simulink model "HevMmPowertrainController"  (R2024a)
settings: configuration reference "VehicleFixed10ms" (kept outside this file)
undefined symbols (not defined in the file): CtrlBcuTrlrBrkGain, CtrlVcuHevMmBattChrgPwrMax, CtrlVcuHevMmBattDischrgPwrMax, CtrlVcuHevMmChrgLmtBpt, CtrlVcuHevMmCSChrgFctr, CtrlVcuHevMmDischrgLmtBpt, CtrlVcuHevMmEngPwr, CtrlVcuHevMmEngSpd, CtrlVcuHevMmEngTrq, CtrlVcuHevMmN_idle, CtrlVcuHevMmRegenBrkCutOff, CtrlVcuHevMmRegenBrkSpdBpt, CtrlVcuHevMmSocBpt, CtrlVcuHevMmSOCChrgFctr, CtrlVcuHevMmSOCmax, CtrlVcuHevMmSOCmin, CtrlVcuHevMmSOCtarget, DiscIntNeverNeededParam, PlntBattChrgMax, PlntBrkActrBoreFrnt, PlntBrkFrntBias, PlntBrkKinFricCffFrnt, PlntBrkNumPadsFrnt, PlntBrkPadMeanRadiusFrnt, PlntBrkPrsFctr, PlntBrkRearBias, PlntDiffrntlRatio, PlntEM1EffTbl, PlntEM1Spd, PlntEM1SpdEff, PlntEM1Trq, PlntEM1TrqEff, PlntEM2EffTbl, PlntEM2Spd, PlntEM2SpdEff, PlntEM2Trq, PlntEM2TrqEff, PlntHevMmGenGearRatio, PlntHevMmMotGearRatio, PlntVehMass, PlntWhlLdRadius
libraries: simulink x15, autolibutils x1
(part 1 of 2)
settings Model: DataDictionary=VirtualVehicleTemplate.sldd  ModifiedByFormat=The MathWorks, Inc.  Creator=The MathWorks, Inc.  LastModifiedBy=The MathWorks, Inc.
settings ConfigSetRef: SourceName=VehicleFixed10ms

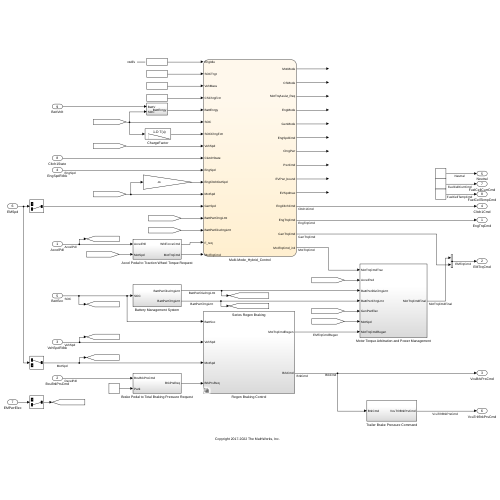
[thumbnail: Simulink's stored preview of the top-level diagram]
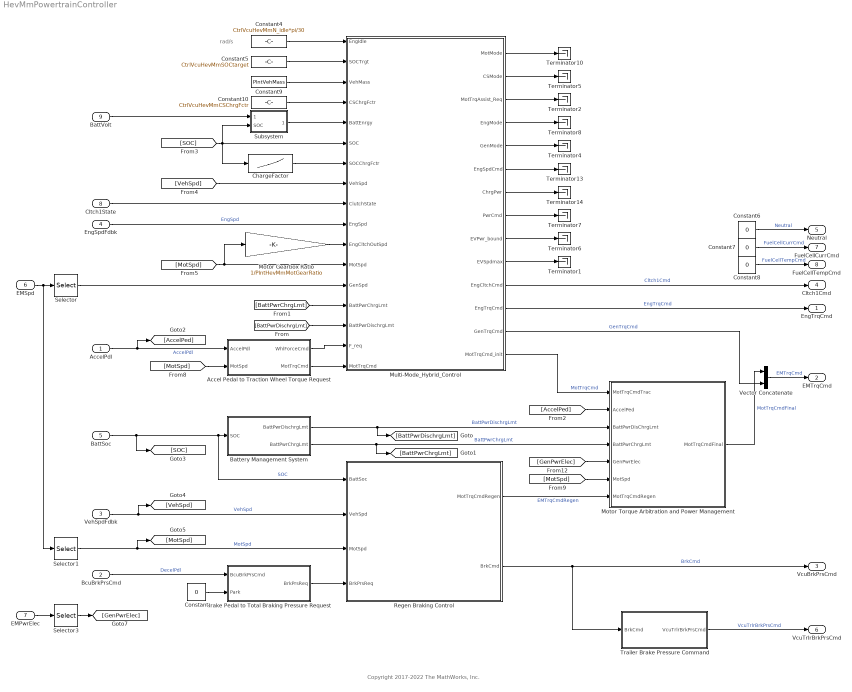
== system HevMmPowertrainController ==
  note: rad/s
  note: Copyright 2017-2022 The MathWorks, Inc.
  AccelPdl : Inport  OutDataTypeStr=double  PortDimensions=1
  BcuBrkPrsCmd : Inport  Port=2  OutDataTypeStr=double  PortDimensions=4
  VehSpdFdbk : Inport  Port=3  OutDataTypeStr=double  PortDimensions=1
  EngSpdFdbk : Inport  Port=4  OutDataTypeStr=double  PortDimensions=1
  BattSoc : Inport  Port=5  OutDataTypeStr=double  PortDimensions=1
  EMSpd : Inport  Port=6  OutDataTypeStr=double  PortDimensions=2
  EMPwrElec : Inport  Port=7  OutDataTypeStr=double  PortDimensions=2
  Cltch1State : Inport  Port=8  OutDataTypeStr=boolean  PortDimensions=1
  BattVolt : Inport  Port=9  OutDataTypeStr=double  PortDimensions=1
  Accel Pedal to Traction Wheel Torque Request : Subsystem  InitFcn=[~]=autosharedicon('autolibinternalvvblock',gcb,0);
  Battery Management System : Subsystem
  Brake Pedal to Total Braking Pressure Request : Subsystem
  ChargeFactor : Lookup_n-D  NumberOfTableDimensions=1  BreakpointsForDimension1=[CtrlVcuHevMmSOCmin CtrlVcuHevMmSOCtarget CtrlVcuHevMmSOCmax]  Table=CtrlVcuHevMmSOCChrgFctr  ExtrapMethod=Clip  UseLastTableValue=on  InternalRulePriority=Speed  RndMeth=Simplest
  Constant{,6..8} (4 alike) : Constant  Value=0  SampleTime=-1
  Constant10 : Constant  Value=CtrlVcuHevMmCSChrgFctr  SampleTime=-1
  Constant4 : Constant  Value=CtrlVcuHevMmN_idle*pi/30  SampleTime=-1
  Constant5 : Constant  Value=CtrlVcuHevMmSOCtarget  SampleTime=-1
  Constant9 : Constant  Value=PlntVehMass  SampleTime=-1
  Motor Gearbox Ratio : Gain  Gain=1/PlntHevMmMotGearRatio
  Motor Torque Arbitration and Power Management : Subsystem
  Multi-Mode_Hybrid_Control : Stateflow chart  TreatAsAtomicUnit=on
  Regen Braking Control : Subsystem  Variant=on  VariantControlMode=label  VariantControl=(default)  LabelModeActiveChoice=Variant
  Selector : Selector  InputPortWidth=2  IndexOptions=Index vector (dialog)  Indices=[2]  OutputSizes=1
  Selector1 : Selector  InputPortWidth=2  IndexOptions=Index vector (dialog)  Indices=[1]  OutputSizes=1
  Selector3 : Selector  InputPortWidth=2  IndexOptions=Index vector (dialog)  Indices=[2]  OutputSizes=1
  Subsystem : Subsystem
  Terminator{1..2,4..8,10,13..14} (10 alike) : Terminator
  Trailer Brake Pressure Command : Subsystem
  Vector Concatenate : Concatenate
  EngTrqCmd : Outport  OutDataTypeStr=double  PortDimensions=1  VectorParamsAs1DForOutWhenUnconnected=off
  EMTrqCmd : Outport  Port=2  OutDataTypeStr=double  PortDimensions=2  VectorParamsAs1DForOutWhenUnconnected=off
  VcuBrkPrsCmd : Outport  Port=3  OutDataTypeStr=double  PortDimensions=4  VectorParamsAs1DForOutWhenUnconnected=off
  Cltch1Cmd : Outport  Port=4  OutDataTypeStr=double  PortDimensions=1  VectorParamsAs1DForOutWhenUnconnected=off
  Neutral : Outport  Port=5  OutDataTypeStr=double  PortDimensions=1  VectorParamsAs1DForOutWhenUnconnected=off
  VcuTrlrBrkPrsCmd : Outport  Port=6  PortDimensions=6  VectorParamsAs1DForOutWhenUnconnected=off
  FuelCellCurrCmd : Outport  Port=7  OutDataTypeStr=double  PortDimensions=1
  FuelCellTempCmd : Outport  Port=8  OutDataTypeStr=double  PortDimensions=1
  wires:
  AccelPdl/1 -> Accel Pedal to Traction Wheel Torque Request/1(AccelPdl), [AccelPed]  "AccelPdl"
  BcuBrkPrsCmd/1 -> Brake Pedal to Total Braking Pressure Request/1(BcuBrkPrsCmd)  "DecelPdl"
  VehSpdFdbk/1 -> [VehSpd], Regen Braking Control/2("VehSpd ")  "VehSpd"
  EngSpdFdbk/1 -> Multi-Mode_Hybrid_Control/10(EngSpd)  "EngSpd"
  BattSoc/1 -> [SOC], Regen Braking Control/1("BattSoc "), Battery Management System/1(SOC)  "SOC"
  Selector1/1 -> [MotSpd], Regen Braking Control/3("MotSpd ")  "MotSpd"
  Battery Management System/2(BattPwrChrgLmt) -> [BattPwrChrgLmt], Motor Torque Arbitration and Power Management/4("BattPwrChrgLmt ")  "BattPwrChrgLmt"
  Battery Management System/1(BattPwrDischrgLmt) -> Motor Torque Arbitration and Power Management/3(BattPwrDisChrgLmt), [BattPwrDischrgLmt]  "BattPwrDischrgLmt"
  [SOC] -> ChargeFactor/1, Subsystem/2(SOC), Multi-Mode_Hybrid_Control/6(SOC)
  [VehSpd] -> Multi-Mode_Hybrid_Control/8(VehSpd)
  Constant4/1 -> Multi-Mode_Hybrid_Control/1(EngIdle)
  Multi-Mode_Hybrid_Control/14(MotTrqCmd_init) -> Motor Torque Arbitration and Power Management/1(MotTrqCmdTrac)  "MotTrqCmd"
  Brake Pedal to Total Braking Pressure Request/1(BrkPrsReq) -> Regen Braking Control/4("BrkPrsReq ")
  Regen Braking Control/1(" MotTrqCmdRegen") -> Motor Torque Arbitration and Power Management/7(MotTrqCmdRegen)  "EMTrqCmdRegen"
  Constant5/1 -> Multi-Mode_Hybrid_Control/2(SOCTrgt)
  ChargeFactor/1 -> Multi-Mode_Hybrid_Control/7(SOCChrgFctr)
  [MotSpd] -> Accel Pedal to Traction Wheel Torque Request/2(MotSpd)
  [AccelPed] -> Motor Torque Arbitration and Power Management/2(AccelPed)
  Selector/1 -> Multi-Mode_Hybrid_Control/13(GenSpd)
  Selector3/1 -> [GenPwrElec]
  EMPwrElec/1 -> Selector3/1
  Motor Torque Arbitration and Power Management/1(MotTrqCmdFinal) -> Vector Concatenate/1  "MotTrqCmdFinal"
  Multi-Mode_Hybrid_Control/13(GenTrqCmd) -> Vector Concatenate/2  "GenTrqCmd"
  Multi-Mode_Hybrid_Control/12(EngTrqCmd) -> EngTrqCmd/1  "EngTrqCmd"
  Constant/1 -> Brake Pedal to Total Braking Pressure Request/2(Park)
  [MotSpd] -> Motor Torque Arbitration and Power Management/6(MotSpd)
  [GenPwrElec] -> Motor Torque Arbitration and Power Management/5(GenPwrElec)
  Vector Concatenate/1 -> EMTrqCmd/1  "EMTrqCmd"
  EMSpd/1 -> Selector1/1, Selector/1
  Constant6/1 -> Neutral/1  "Neutral"
  Multi-Mode_Hybrid_Control/11(EngCltchCmd) -> Cltch1Cmd/1  "Cltch1Cmd"
  Constant7/1 -> FuelCellCurrCmd/1  "FuelCellCurrCmd"
  Constant8/1 -> FuelCellTempCmd/1  "FuelCellTempCmd"
  Multi-Mode_Hybrid_Control/7(ChrgPwr) -> Terminator14/1
  Multi-Mode_Hybrid_Control/8(PwrCmd) -> Terminator7/1
  Multi-Mode_Hybrid_Control/9(EVPwr_bound) -> Terminator6/1
  Multi-Mode_Hybrid_Control/10(EVSpdmax) -> Terminator1/1
  Multi-Mode_Hybrid_Control/6(EngSpdCmd) -> Terminator13/1
  Multi-Mode_Hybrid_Control/5(GenMode) -> Terminator4/1
  Multi-Mode_Hybrid_Control/4(EngMode) -> Terminator8/1
  Multi-Mode_Hybrid_Control/3(MotTrqAssist_Req) -> Terminator2/1
  Multi-Mode_Hybrid_Control/2(CSMode) -> Terminator5/1
  Multi-Mode_Hybrid_Control/1(MotMode) -> Terminator10/1
  [BattPwrChrgLmt] -> Multi-Mode_Hybrid_Control/14(BattPwrChrgLmt)
  [BattPwrDischrgLmt] -> Multi-Mode_Hybrid_Control/15(BattPwrDischrgLmt)
  [MotSpd] -> Motor Gearbox Ratio/1, Multi-Mode_Hybrid_Control/12(MotSpd)
  Cltch1State/1 -> Multi-Mode_Hybrid_Control/9(ClutchState)
  Motor Gearbox Ratio/1 -> Multi-Mode_Hybrid_Control/11(EngCltchOutSpd)
  Constant9/1 -> Multi-Mode_Hybrid_Control/3(VehMass)
  Constant10/1 -> Multi-Mode_Hybrid_Control/4(CSChrgFctr)
  Subsystem/1(BattEnrgy) -> Multi-Mode_Hybrid_Control/5(BattEnrgy)
  BattVolt/1 -> Subsystem/1(BattV)
  Accel Pedal to Traction Wheel Torque Request/2(MotTrqCmd) -> Multi-Mode_Hybrid_Control/17(MotTrqCmd)
  Accel Pedal to Traction Wheel Torque Request/1(WhlForceCmd) -> Multi-Mode_Hybrid_Control/16(F_req)
  Regen Braking Control/2(" BrkCmd") -> Trailer Brake Pressure Command/1(BrkCmd), VcuBrkPrsCmd/1  "BrkCmd"
  Trailer Brake Pressure Command/1(VcuTrlrBrkPrsCmd) -> VcuTrlrBrkPrsCmd/1  "VcuTrlrBrkPrsCmd"

== system HevMmPowertrainController/Accel Pedal to Traction Wheel Torque Request ==
  AccelPdl : Inport
  MotSpd : Inport  Port=2
  MaxMotTrqVsSpd : Lookup_n-D  NumberOfTableDimensions=1  BreakpointsForDimension1=PlntEM1Spd*30/pi  Table=PlntEM1Trq  ExtrapMethod=Clip  UseLastTableValue=on  InternalRulePriority=Speed  OutDataTypeStr=Inherit: Inherit from 'Table data'  RndMeth=Simplest
  MotTrq_to_WhlForce : Gain  Gain=(PlntDiffrntlRatio*PlntHevMmMotGearRatio)/PlntWhlLdRadius
  Product1 : Product
  rads_to_rpm : Gain  Gain=30/pi
  WhlForceCmd : Outport  VectorParamsAs1DForOutWhenUnconnected=off
  MotTrqCmd : Outport  Port=2  VectorParamsAs1DForOutWhenUnconnected=off
  wires:
  Product1/1 -> MotTrqCmd/1, MotTrq_to_WhlForce/1
  MaxMotTrqVsSpd/1 -> Product1/2
  AccelPdl/1 -> Product1/1
  rads_to_rpm/1 -> MaxMotTrqVsSpd/1
  MotSpd/1 -> rads_to_rpm/1
  MotTrq_to_WhlForce/1 -> WhlForceCmd/1

== system HevMmPowertrainController/Battery Management System ==
  note: Limit battery charge / discharge power based on SOC
  SOC : Inport
  ChrgLmt : Lookup_n-D  NumberOfTableDimensions=1  BreakpointsForDimension1=CtrlVcuHevMmSocBpt  Table=CtrlVcuHevMmChrgLmtBpt  ExtrapMethod=Clip  UseLastTableValue=on  InternalRulePriority=Speed  RndMeth=Simplest
  DischrgLmt : Lookup_n-D  NumberOfTableDimensions=1  BreakpointsForDimension1=CtrlVcuHevMmSocBpt  Table=CtrlVcuHevMmDischrgLmtBpt  ExtrapMethod=Clip  UseLastTableValue=on  InternalRulePriority=Speed  RndMeth=Simplest
  MaxChrg : Constant  Value=CtrlVcuHevMmBattChrgPwrMax  SampleTime=-1
  MaxDischrg : Constant  Value=CtrlVcuHevMmBattDischrgPwrMax  SampleTime=-1
  Product : Product
  Product1 : Product
  BattPwrDischrgLmt : Outport  VectorParamsAs1DForOutWhenUnconnected=off
  BattPwrChrgLmt : Outport  Port=2  VectorParamsAs1DForOutWhenUnconnected=off
  wires:
  SOC/1 -> DischrgLmt/1, ChrgLmt/1
  MaxChrg/1 -> Product1/2
  MaxDischrg/1 -> Product/2
  Product/1 -> BattPwrDischrgLmt/1
  Product1/1 -> BattPwrChrgLmt/1
  ChrgLmt/1 -> Product1/1
  DischrgLmt/1 -> Product/1

== system HevMmPowertrainController/Brake Pedal to Total Braking Pressure Request ==
  BcuBrkPrsCmd : Inport
  Park : Inport  Port=2
  Front Bias : Constant  Value=PlntBrkFrntBias  SampleTime=-1
  Gain4 : Gain  Gain=PlntBrkPrsFctr
  Mux : Mux
  Product : Product
  Rear Bias : Constant  Value=PlntBrkRearBias  SampleTime=-1
  Terminator : Terminator
  BrkPrsReq : Outport  VectorParamsAs1DForOutWhenUnconnected=off
  wires:
  BcuBrkPrsCmd/1 -> Product/2
  Mux/1 -> Product/1
  Rear Bias/1 -> Mux/4, Mux/3
  Front Bias/1 -> Mux/1, Mux/2
  Gain4/1 -> BrkPrsReq/1
  Product/1 -> Gain4/1
  Park/1 -> Terminator/1

== system HevMmPowertrainController/Motor Torque Arbitration and Power Management ==
  MotTrqCmdTrac : Inport
  AccelPed : Inport  Port=2
  BattPwrDisChrgLmt : Inport  Port=3
  "BattPwrChrgLmt " : Inport  Port=4
  GenPwrElec : Inport  Port=5
  MotSpd : Inport  Port=6
  MotTrqCmdRegen : Inport  Port=7
  Accel Decel Switch : Switch  Criteria=u2 > Threshold  SaturateOnIntegerOverflow=off  InputSameDT=off
  Compare To Constant : simulink/Logic and Bit Operations/Compare To Constant  relop=>  const=0  OutDataTypeStr=boolean
  Power Management : Subsystem
  MotTrqCmdFinal : Outport  VectorParamsAs1DForOutWhenUnconnected=off
  wires:
  AccelPed/1 -> Compare To Constant/1
  MotTrqCmdRegen/1 -> Accel Decel Switch/3
  Compare To Constant/1 -> Accel Decel Switch/2
  MotTrqCmdTrac/1 -> Accel Decel Switch/1
  Power Management/1(MotTrqLim) -> MotTrqCmdFinal/1
  Accel Decel Switch/1 -> Power Management/5(MotTrqCmd)
  BattPwrDisChrgLmt/1 -> Power Management/1(BattPwrDischrgLmt)
  GenPwrElec/1 -> Power Management/2(GenPwrElec)
  "BattPwrChrgLmt "/1 -> Power Management/3(BattPwrChrgLmt)
  MotSpd/1 -> Power Management/4(MotSpd)

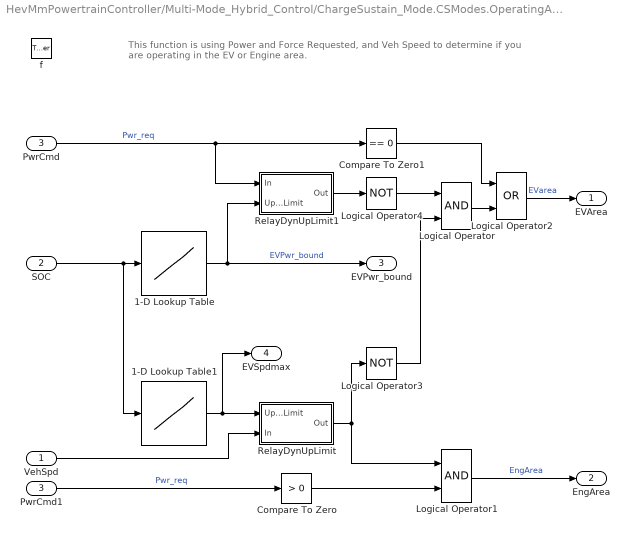
== system HevMmPowertrainController/Multi-Mode_Hybrid_Control/ChargeSustain_Mode.CSModes.OperatingAreaCalc ==
  note: This function is using Power and Force Requested, and Veh Speed to determine
      | if you are operating in the EV or Engine area.
  VehSpd : Inport  PortDimensions=1
  SOC : Inport  Port=2  PortDimensions=1
  PwrCmd : Inport  Port=3
  f : TriggerPort  TriggerType=function-call  VariantControl=Variant  StatesWhenEnabling=reset
      settings: CopyFcn=Stateflow.SLINSF.SimulinkMan.removeBlockPreDeleteFcn  PreDeleteFcn=Stateflow.SLINSF.SimulinkMan.unsafePredeleteFcn
  1-D Lookup Table : Lookup_n-D  NumberOfTableDimensions=1  BreakpointsForDimension1=[CtrlVcuHevMmSOCmin CtrlVcuHevMmSOCtarget CtrlVcuHevMmSOCmax]  Table=[0 CtrlVcuHevMmEngPwr(4) CtrlVcuHevMmBattDischrgPwrMax]  ExtrapMethod=Clip  UseLastTableValue=on  InternalRulePriority=Speed  RndMeth=Simplest
  1-D Lookup Table1 : Lookup_n-D  NumberOfTableDimensions=1  BreakpointsForDimension1=[CtrlVcuHevMmSOCtarget CtrlVcuHevMmSOCmax]  Table=[24.6 33.5]  ExtrapMethod=Clip  UseLastTableValue=on  InternalRulePriority=Speed  RndMeth=Simplest
  Compare To Zero : simulink/Logic and Bit Operations/Compare To Zero  relop=>  OutDataTypeStr=boolean
  Compare To Zero1 : simulink/Logic and Bit Operations/Compare To Zero  relop===  OutDataTypeStr=boolean
  Logical Operator : Logic  AllPortsSameDT=off  OutDataTypeStr=boolean
  Logical Operator1 : Logic  AllPortsSameDT=off  OutDataTypeStr=boolean
  Logical Operator2 : Logic  Operator=OR  AllPortsSameDT=off  OutDataTypeStr=boolean
  Logical Operator3 : Logic  Operator=NOT  AllPortsSameDT=off  OutDataTypeStr=boolean
  Logical Operator4 : Logic  Operator=NOT  AllPortsSameDT=off  OutDataTypeStr=boolean
  PwrCmd1 : InportShadow  Port=3
  RelayDynUpLimit : Subsystem
  RelayDynUpLimit1 : Subsystem
  EVArea : Outport  VectorParamsAs1DForOutWhenUnconnected=off
  EngArea : Outport  Port=2  VectorParamsAs1DForOutWhenUnconnected=off
  EVPwr_bound : Outport  Port=3  VectorParamsAs1DForOutWhenUnconnected=off
  EVSpdmax : Outport  Port=4  VectorParamsAs1DForOutWhenUnconnected=off
  wires:
  Logical Operator1/1 -> EngArea/1  "EngArea"
  Logical Operator/1 -> Logical Operator2/2
  Logical Operator3/1 -> Logical Operator/2
  VehSpd/1 -> RelayDynUpLimit/2(In)
  1-D Lookup Table1/1 -> EVSpdmax/1, RelayDynUpLimit/1(Upper Limit)
  PwrCmd/1 -> RelayDynUpLimit1/1(In), Compare To Zero1/1  "Pwr_req"
  Compare To Zero1/1 -> Logical Operator2/1
  Logical Operator2/1 -> EVArea/1  "EVarea"
  1-D Lookup Table/1 -> RelayDynUpLimit1/2(Upper Limit), EVPwr_bound/1  "EVPwr_bound"
  SOC/1 -> 1-D Lookup Table/1, 1-D Lookup Table1/1
  Compare To Zero/1 -> Logical Operator1/2
  PwrCmd1/1 -> Compare To Zero/1  "Pwr_req"
  RelayDynUpLimit/1(Out) -> Logical Operator1/1, Logical Operator3/1
  RelayDynUpLimit1/1(Out) -> Logical Operator4/1
  Logical Operator4/1 -> Logical Operator/1

== system HevMmPowertrainController/Multi-Mode_Hybrid_Control/ChargeSustain_Mode.Engine_Control.Eng.Clutch_Close.ClutchControl ==
  note: When error is <=5 rads/s
      | clutch commanded closed
  EngCltchOutSpd : Inport
  EngSpd : Inport  Port=2
  f : TriggerPort  TriggerType=function-call  VariantControl=Variant  StatesWhenEnabling=reset  SampleTime=-1
      settings: CopyFcn=Stateflow.SLINSF.SimulinkMan.removeBlockPreDeleteFcn  PreDeleteFcn=Stateflow.SLINSF.SimulinkMan.unsafePredeleteFcn
  Abs1 : Abs  SaturateOnIntegerOverflow=off
  Compare To Constant1 : simulink/Logic and Bit Operations/Compare To Constant  relop=<=  const=5  OutDataTypeStr=boolean
  Subtract2 : Sum  Inputs=+-
  EngCltchCmd : Outport  VectorParamsAs1DForOutWhenUnconnected=off
  wires:
  EngCltchOutSpd/1 -> Subtract2/1
  Abs1/1 -> Compare To Constant1/1
  EngSpd/1 -> Subtract2/2
  Subtract2/1 -> Abs1/1
  Compare To Constant1/1 -> EngCltchCmd/1

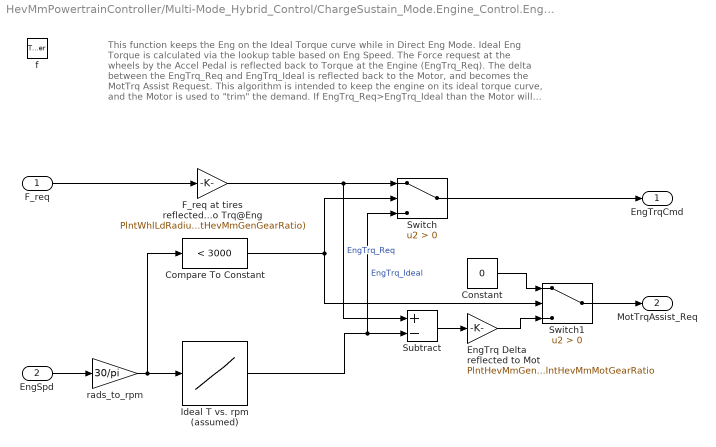
== system HevMmPowertrainController/Multi-Mode_Hybrid_Control/ChargeSustain_Mode.Engine_Control.Eng.Direct_Engine_Drive.EngTrqControl ==
  note: This function keeps the Eng on the Ideal Torque curve while in Direct Eng Mode.
      | Ideal Eng Torque is calculated via the lookup table based on Eng Speed.
      | The Force request at the wheels by the Accel Pedal is reflected back to Torque at
      | the Engine (EngTrq_Req).  The delta between the EngTrq_Req and EngTrq_Ideal
      | is reflected back to the Motor, and becomes the MotTrq Assist Request.  This algorithm
      | is intended to keep the engine on its ideal torque curve, and the Motor is used to "trim"
      | the demand.  If EngTrq_Req>EngTrq_Ideal than the Motor will provide assistance in
      | traction.  If EngTrq_Req<EngTrq_Ideal, the Motor will provide assistance through regen.
  F_req : Inport
  EngSpd : Inport  Port=2
  f : TriggerPort  TriggerType=function-call  VariantControl=Variant  StatesWhenEnabling=reset  SampleTime=-1
      settings: CopyFcn=Stateflow.SLINSF.SimulinkMan.removeBlockPreDeleteFcn  PreDeleteFcn=Stateflow.SLINSF.SimulinkMan.unsafePredeleteFcn
  Compare To Constant : simulink/Logic and Bit Operations/Compare To Constant  relop=<  const=3000  OutDataTypeStr=boolean
  Constant : Constant  Value=0  SampleTime=-1
  EngTrq Delta reflected to Mot : Gain  Gain=PlntHevMmGenGearRatio/PlntHevMmMotGearRatio
  F_req at tires reflected back to Trq@Eng : Gain  Gain=PlntWhlLdRadius/(PlntDiffrntlRatio*PlntHevMmGenGearRatio)
  Ideal T vs. rpm (assumed) : Lookup_n-D  NumberOfTableDimensions=1  BreakpointsForDimension1=CtrlVcuHevMmEngSpd  BreakpointsForDimension1DataTypeStr=Inherit: Inherit from 'Breakpoint data'  Table=CtrlVcuHevMmEngTrq  TableDataTypeStr=Inherit: Inherit from 'Table data'  ExtrapMethod=Clip  UseLastTableValue=on  InternalRulePriority=Speed  OutDataTypeStr=single  RndMeth=Simplest
  Subtract : Sum  Inputs=+-
  Switch : Switch  Criteria=u2 > Threshold  SaturateOnIntegerOverflow=off  InputSameDT=off
  Switch1 : Switch  Criteria=u2 > Threshold  SaturateOnIntegerOverflow=off  InputSameDT=off
  rads_to_rpm : Gain  Gain=30/pi
  EngTrqCmd : Outport  VectorParamsAs1DForOutWhenUnconnected=off
  MotTrqAssist_Req : Outport  Port=2  VectorParamsAs1DForOutWhenUnconnected=off
  wires:
  F_req/1 -> F_req at tires reflected back to Trq@Eng/1
  F_req at tires reflected back to Trq@Eng/1 -> Switch/1, Subtract/1  "EngTrq_Req"
  Subtract/1 -> EngTrq Delta reflected to Mot/1
  Ideal T vs. rpm (assumed)/1 -> Subtract/2, Switch/3  "EngTrq_Ideal"
  rads_to_rpm/1 -> Compare To Constant/1, Ideal T vs. rpm (assumed)/1
  EngSpd/1 -> rads_to_rpm/1
  Compare To Constant/1 -> Switch1/2, Switch/2
  EngTrq Delta reflected to Mot/1 -> Switch1/3
  Constant/1 -> Switch1/1
  Switch/1 -> EngTrqCmd/1
  Switch1/1 -> MotTrqAssist_Req/1

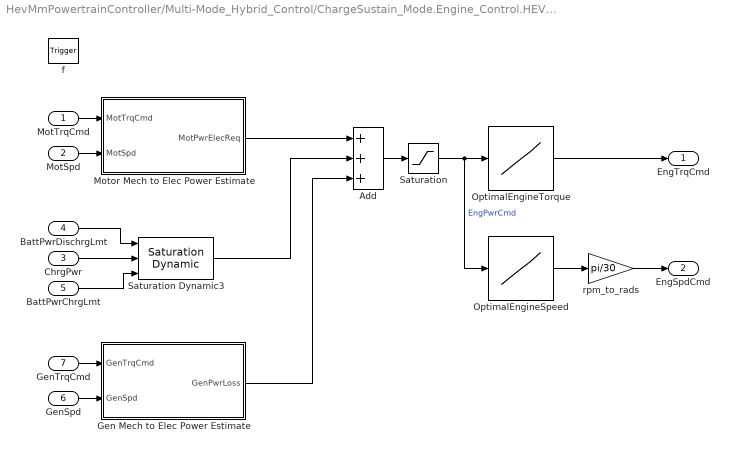
== system HevMmPowertrainController/Multi-Mode_Hybrid_Control/ChargeSustain_Mode.Engine_Control.HEV.TrqCalc ==
  MotTrqCmd : Inport
  MotSpd : Inport  Port=2
  ChrgPwr : Inport  Port=3
  BattPwrDischrgLmt : Inport  Port=4
  BattPwrChrgLmt : Inport  Port=5
  GenSpd : Inport  Port=6
  GenTrqCmd : Inport  Port=7
  f : TriggerPort  TriggerType=function-call  VariantControl=Variant  StatesWhenEnabling=reset
      settings: CopyFcn=Stateflow.SLINSF.SimulinkMan.removeBlockPreDeleteFcn  PreDeleteFcn=Stateflow.SLINSF.SimulinkMan.unsafePredeleteFcn
  Add : Sum  Inputs=+++
  Gen Mech to Elec Power Estimate : Subsystem
  Motor Mech to Elec Power Estimate : Subsystem
  OptimalEngineSpeed : Lookup_n-D  NumberOfTableDimensions=1  BreakpointsForDimension1=CtrlVcuHevMmEngPwr  Table=CtrlVcuHevMmEngSpd  ExtrapMethod=Clip  UseLastTableValue=on  InternalRulePriority=Speed  RndMeth=Simplest
  OptimalEngineTorque : Lookup_n-D  NumberOfTableDimensions=1  BreakpointsForDimension1=CtrlVcuHevMmEngPwr  Table=CtrlVcuHevMmEngTrq  ExtrapMethod=Clip  UseLastTableValue=on  InternalRulePriority=Speed  RndMeth=Simplest
  Saturation : Saturate  UpperLimit=inf  LowerLimit=0
  Saturation Dynamic3 : simulink/Discontinuities/Saturation Dynamic  OutMin=[]  OutMax=[]  OutDataTypeStr=Inherit: Same as second input  OutDataType=fixdt(1, 16)  OutScaling=2^-10  DoSatur=off
  rpm_to_rads : Gain  Gain=pi/30
  EngTrqCmd : Outport  VectorParamsAs1DForOutWhenUnconnected=off
  EngSpdCmd : Outport  Port=2  VectorParamsAs1DForOutWhenUnconnected=off
  wires:
  rpm_to_rads/1 -> EngSpdCmd/1
  OptimalEngineSpeed/1 -> rpm_to_rads/1
  Saturation/1 -> OptimalEngineTorque/1, OptimalEngineSpeed/1  "EngPwrCmd"
  MotTrqCmd/1 -> Motor Mech to Elec Power Estimate/1(MotTrqCmd)
  MotSpd/1 -> Motor Mech to Elec Power Estimate/2(MotSpd)
  Motor Mech to Elec Power Estimate/1(MotPwrElecReq) -> Add/1
  Add/1 -> Saturation/1
  ChrgPwr/1 -> Saturation Dynamic3/2
  BattPwrChrgLmt/1 -> Saturation Dynamic3/3
  Saturation Dynamic3/1 -> Add/2
  BattPwrDischrgLmt/1 -> Saturation Dynamic3/1
  OptimalEngineTorque/1 -> EngTrqCmd/1
  GenSpd/1 -> Gen Mech to Elec Power Estimate/2(GenSpd)
  GenTrqCmd/1 -> Gen Mech to Elec Power Estimate/1(GenTrqCmd)
  Gen Mech to Elec Power Estimate/1(GenPwrLoss) -> Add/3

== system HevMmPowertrainController/Multi-Mode_Hybrid_Control/ChargeSustain_Mode.Generator_Control.On.GenControl ==
  EngSpd : Inport
  EngSpdCmd : Inport  Port=2
  f : TriggerPort  TriggerType=function-call  VariantControl=Variant  StatesWhenEnabling=reset  SampleTime=-1
      settings: CopyFcn=Stateflow.SLINSF.SimulinkMan.removeBlockPreDeleteFcn  PreDeleteFcn=Stateflow.SLINSF.SimulinkMan.unsafePredeleteFcn
  State-Feedback Controller : Subsystem
  Torque Limit : Subsystem
  GenTrqCmd : Outport  VectorParamsAs1DForOutWhenUnconnected=off
  wires:
  EngSpd/1 -> State-Feedback Controller/2(y), Torque Limit/2(GenSpd)
  EngSpdCmd/1 -> State-Feedback Controller/1(r)
  Torque Limit/1(GenTrqCmd) -> GenTrqCmd/1
  State-Feedback Controller/1(Out1) -> Torque Limit/1(GenTrq)

== system HevMmPowertrainController/Regen Braking Control ==
  "BattSoc " : Inport
  "VehSpd " : Inport  Port=2
  "MotSpd " : Inport  Port=3
  "BrkPrsReq " : Inport  Port=4
  Parallel Regen Braking : Subsystem  InitFcn=[~]=autosharedicon('autolibinternalvvblock',gcb,0);  VariantControl=(default)
  Series Regen Braking : Subsystem  InitFcn=[~]=autosharedicon('autolibinternalvvblock',gcb,0);  VariantControl=Variant
  " MotTrqCmdRegen" : Outport  VectorParamsAs1DForOutWhenUnconnected=off
  " BrkCmd" : Outport  Port=2  VectorParamsAs1DForOutWhenUnconnected=off

== system HevMmPowertrainController/Subsystem ==
  BattV : Inport
  SOC : Inport  Port=2
  BattCap_As : Constant  Value=PlntBattChrgMax*3600  SampleTime=-1
  Gain1 : Gain  Gain=1/100
  Product : Product  Inputs=3
  BattEnrgy : Outport  VectorParamsAs1DForOutWhenUnconnected=off
  wires:
  SOC/1 -> Gain1/1
  BattCap_As/1 -> Product/1
  Product/1 -> BattEnrgy/1
  BattV/1 -> Product/2
  Gain1/1 -> Product/3

== system HevMmPowertrainController/Trailer Brake Pressure Command ==
  BrkCmd : Inport
  Gain1 : Gain  Gain=CtrlBcuTrlrBrkGain
  Probe : Probe  ProbeSampleTime=off  ProbeComplexSignal=off
  Product : Product  Inputs=*/
  Selector2 : Selector  InputPortWidth=1  IndexOptions=Index vector (dialog)  Indices=[1 1 1 1 1 1]  OutputSizes=1
  Sum : Sum  Inputs=+
  VcuTrlrBrkPrsCmd : Outport
  wires:
  Gain1/1 -> Selector2/1
  Product/1 -> Gain1/1
  Probe/1 -> Product/2
  BrkCmd/1 -> Probe/1, Sum/1
  Sum/1 -> Product/1
  Selector2/1 -> VcuTrlrBrkPrsCmd/1

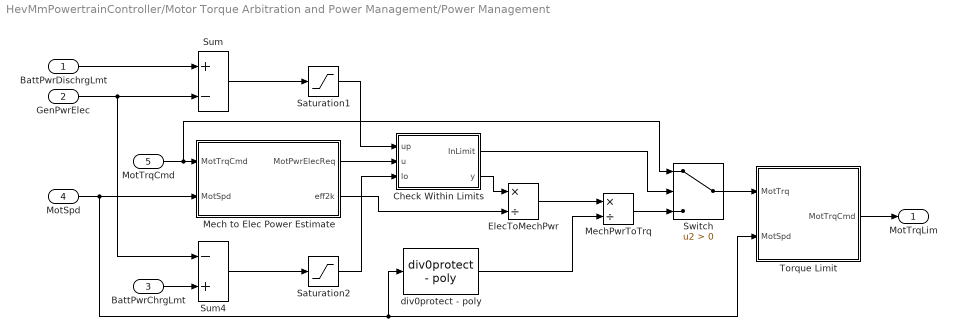
== system HevMmPowertrainController/Motor Torque Arbitration and Power Management/Power Management ==
  BattPwrDischrgLmt : Inport
  GenPwrElec : Inport  Port=2
  BattPwrChrgLmt : Inport  Port=3
  MotSpd : Inport  Port=4
  MotTrqCmd : Inport  Port=5
  Check Within Limits : Subsystem
  ElecToMechPwr : Product  Inputs=*/
  Mech to Elec Power Estimate : Subsystem
  MechPwrToTrq : Product  Inputs=*/
  Saturation1 : Saturate  UpperLimit=inf  LowerLimit=0
  Saturation2 : Saturate  UpperLimit=0  LowerLimit=-inf
  Sum : Sum  Inputs=+-
  Sum4 : Sum  Inputs=-+
  Switch : Switch  Criteria=u2 > Threshold  SaturateOnIntegerOverflow=off  InputSameDT=off
  Torque Limit : Subsystem
  div0protect - poly : autolibutils/div0protect - poly  thresh=2  ZeroCross1=off  aMode=aMode
  MotTrqLim : Outport  VectorParamsAs1DForOutWhenUnconnected=off
  wires:
  BattPwrChrgLmt/1 -> Sum4/2
  Sum4/1 -> Saturation2/1
  Sum/1 -> Saturation1/1
  GenPwrElec/1 -> Sum/2, Sum4/1
  BattPwrDischrgLmt/1 -> Sum/1
  MotSpd/1 -> Torque Limit/2(MotSpd), div0protect - poly/1, Mech to Elec Power Estimate/2(MotSpd)
  MotTrqCmd/1 -> Switch/1, Mech to Elec Power Estimate/1(MotTrqCmd)
  div0protect - poly/1 -> MechPwrToTrq/2
  Mech to Elec Power Estimate/2(eff2k) -> ElecToMechPwr/2
  ElecToMechPwr/1 -> MechPwrToTrq/1
  MechPwrToTrq/1 -> Switch/3
  Torque Limit/1(MotTrqCmd) -> MotTrqLim/1
  Saturation1/1 -> Check Within Limits/1(up)
  Mech to Elec Power Estimate/1(MotPwrElecReq) -> Check Within Limits/2(u)
  Saturation2/1 -> Check Within Limits/3(lo)
  Check Within Limits/2(y) -> ElecToMechPwr/1
  Switch/1 -> Torque Limit/1(MotTrq)
  Check Within Limits/1(InLimit) -> Switch/2

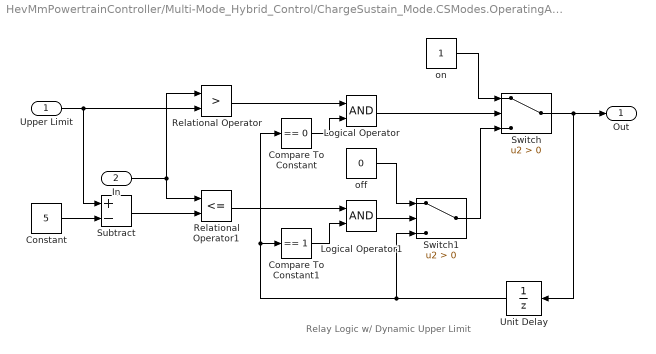
== system HevMmPowertrainController/Multi-Mode_Hybrid_Control/ChargeSustain_Mode.CSModes.OperatingAreaCalc/RelayDynUpLimit ==
  note: Relay Logic w/ Dynamic Upper Limit
  Upper Limit : Inport
  In : Inport  Port=2
  Compare To Constant : simulink/Logic and Bit Operations/Compare To Constant  relop===  const=0  OutDataTypeStr=boolean
  Compare To Constant1 : simulink/Logic and Bit Operations/Compare To Constant  relop===  const=1  OutDataTypeStr=boolean
  Constant : Constant  Value=5
  Logical Operator : Logic  AllPortsSameDT=off  OutDataTypeStr=boolean
  Logical Operator1 : Logic  AllPortsSameDT=off  OutDataTypeStr=boolean
  Relational Operator : RelationalOperator  Operator=>  OutDataTypeStr=boolean  RndMeth=Simplest  InputSameDT=off
  Relational Operator1 : RelationalOperator  Operator=<=  OutDataTypeStr=boolean  RndMeth=Simplest  InputSameDT=off
  Subtract : Sum  Inputs=+-
  Switch : Switch  Criteria=u2 > Threshold  SaturateOnIntegerOverflow=off  InputSameDT=off
  Switch1 : Switch  Criteria=u2 > Threshold  SaturateOnIntegerOverflow=off  InputSameDT=off
  Unit Delay : UnitDelay  SampleTime=-1  HasFrameUpgradeWarning=on
  off : Constant  Value=0  OutDataTypeStr=boolean
  on : Constant  OutDataTypeStr=boolean
  Out : Outport  VectorParamsAs1DForOutWhenUnconnected=off
  wires:
  In/1 -> Relational Operator1/1, Relational Operator/1
  Upper Limit/1 -> Subtract/1, Relational Operator/2
  Subtract/1 -> Relational Operator1/2
  Relational Operator/1 -> Logical Operator/1
  Compare To Constant/1 -> Logical Operator/2
  Relational Operator1/1 -> Logical Operator1/1
  Compare To Constant1/1 -> Logical Operator1/2
  Logical Operator/1 -> Switch/2
  on/1 -> Switch/1
  Logical Operator1/1 -> Switch1/2
  off/1 -> Switch1/1
  Switch1/1 -> Switch/3
  Switch/1 -> Unit Delay/1, Out/1
  Unit Delay/1 -> Switch1/3, Compare To Constant/1, Compare To Constant1/1
  Constant/1 -> Subtract/2

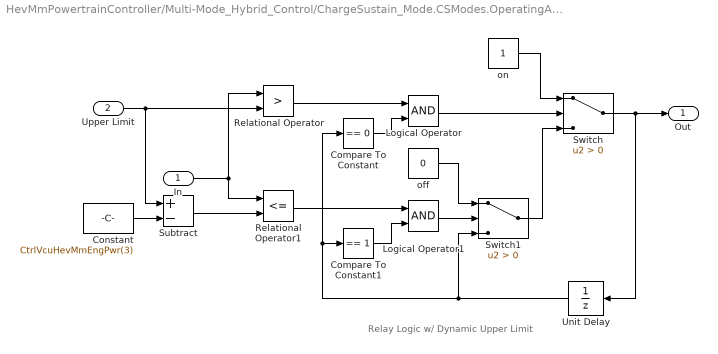
== system HevMmPowertrainController/Multi-Mode_Hybrid_Control/ChargeSustain_Mode.CSModes.OperatingAreaCalc/RelayDynUpLimit1 ==
  note: Relay Logic w/ Dynamic Upper Limit
  In : Inport
  Upper Limit : Inport  Port=2
  Compare To Constant : simulink/Logic and Bit Operations/Compare To Constant  relop===  const=0  OutDataTypeStr=boolean
  Compare To Constant1 : simulink/Logic and Bit Operations/Compare To Constant  relop===  const=1  OutDataTypeStr=boolean
  Constant : Constant  Value=CtrlVcuHevMmEngPwr(3)
  Logical Operator : Logic  AllPortsSameDT=off  OutDataTypeStr=boolean
  Logical Operator1 : Logic  AllPortsSameDT=off  OutDataTypeStr=boolean
  Relational Operator : RelationalOperator  Operator=>  OutDataTypeStr=boolean  RndMeth=Simplest  InputSameDT=off
  Relational Operator1 : RelationalOperator  Operator=<=  OutDataTypeStr=boolean  RndMeth=Simplest  InputSameDT=off
  Subtract : Sum  Inputs=+-
  Switch : Switch  Criteria=u2 > Threshold  SaturateOnIntegerOverflow=off  InputSameDT=off
  Switch1 : Switch  Criteria=u2 > Threshold  SaturateOnIntegerOverflow=off  InputSameDT=off
  Unit Delay : UnitDelay  SampleTime=-1  HasFrameUpgradeWarning=on
  off : Constant  Value=0  OutDataTypeStr=boolean
  on : Constant  OutDataTypeStr=boolean
  Out : Outport  VectorParamsAs1DForOutWhenUnconnected=off
  wires:
  Constant/1 -> Subtract/2
  Unit Delay/1 -> Compare To Constant1/1, Compare To Constant/1, Switch1/3
  Switch/1 -> Out/1, Unit Delay/1
  Switch1/1 -> Switch/3
  off/1 -> Switch1/1
  Logical Operator1/1 -> Switch1/2
  on/1 -> Switch/1
  Logical Operator/1 -> Switch/2
  Compare To Constant1/1 -> Logical Operator1/2
  Relational Operator1/1 -> Logical Operator1/1
  Compare To Constant/1 -> Logical Operator/2
  Relational Operator/1 -> Logical Operator/1
  Subtract/1 -> Relational Operator1/2
  Upper Limit/1 -> Relational Operator/2, Subtract/1
  In/1 -> Relational Operator/1, Relational Operator1/1

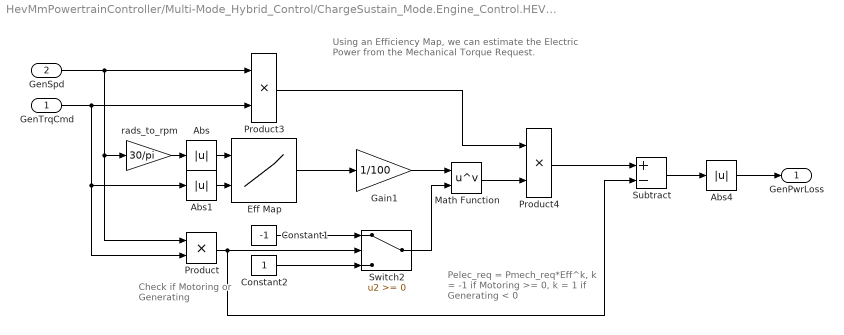
== system HevMmPowertrainController/Multi-Mode_Hybrid_Control/ChargeSustain_Mode.Engine_Control.HEV.TrqCalc/Gen Mech to Elec Power Estimate ==
  note: Pelec_req = Pmech_req*Eff^k,
      | k = -1 if Motoring >= 0,
      | k = 1 if Generating < 0
  note: Using an Efficiency Map, we can estimate the
      | Electric Power from the Mechanical  Torque Request.
  note: Check if Motoring
      | or Generating
  GenTrqCmd : Inport
  GenSpd : Inport  Port=2
  Abs : Abs  SaturateOnIntegerOverflow=off
  Abs1 : Abs  SaturateOnIntegerOverflow=off
  Abs4 : Abs  SaturateOnIntegerOverflow=off
  Constant1 : Constant  Value=-1  SampleTime=-1
  Constant2 : Constant  SampleTime=-1
  Eff Map : Lookup_n-D  BreakpointsForDimension1=PlntEM2SpdEff*30/pi  BreakpointsForDimension2=PlntEM2TrqEff  Table=PlntEM2EffTbl  ExtrapMethod=Clip  UseLastTableValue=on  InternalRulePriority=Speed  OutDataTypeStr=Inherit: Inherit from 'Table data'  RndMeth=Simplest
      settings: InputPortMap=u0,u1
  Gain1 : Gain  Gain=1/100
  Math Function : Math  Operator=pow  SignedPower=on  OutputSignalType=real
  Product : Product
  Product3 : Product
  Product4 : Product
  Subtract : Sum  Inputs=+-
  Switch2 : Switch  SaturateOnIntegerOverflow=off  InputSameDT=off
  rads_to_rpm : Gain  Gain=30/pi
  GenPwrLoss : Outport  VectorParamsAs1DForOutWhenUnconnected=off
  wires:
  GenTrqCmd/1 -> Abs1/1, Product/2, Product3/2
  GenSpd/1 -> rads_to_rpm/1, Product/1, Product3/1
  rads_to_rpm/1 -> Abs/1
  Abs1/1 -> Eff Map/2
  Math Function/1 -> Product4/2
  Gain1/1 -> Math Function/1
  Abs/1 -> Eff Map/1
  Eff Map/1 -> Gain1/1
  Constant2/1 -> Switch2/3
  Constant1/1 -> Switch2/1
  Switch2/1 -> Math Function/2
  Product3/1 -> Product4/1
  Product/1 -> Subtract/2, Switch2/2
  Product4/1 -> Subtract/1
  Subtract/1 -> Abs4/1
  Abs4/1 -> GenPwrLoss/1

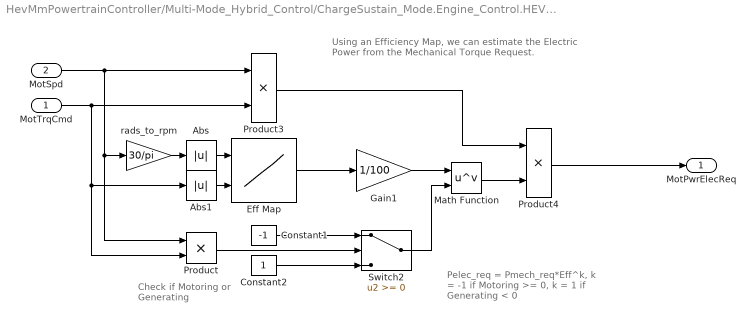
== system HevMmPowertrainController/Multi-Mode_Hybrid_Control/ChargeSustain_Mode.Engine_Control.HEV.TrqCalc/Motor Mech to Elec Power Estimate ==
  note: Check if Motoring
      | or Generating
  note: Using an Efficiency Map, we can estimate the
      | Electric Power from the Mechanical  Torque Request.
  note: Pelec_req = Pmech_req*Eff^k,
      | k = -1 if Motoring >= 0,
      | k = 1 if Generating < 0
  MotTrqCmd : Inport
  MotSpd : Inport  Port=2
  Abs : Abs  SaturateOnIntegerOverflow=off
  Abs1 : Abs  SaturateOnIntegerOverflow=off
  Constant1 : Constant  Value=-1  SampleTime=-1
  Constant2 : Constant  SampleTime=-1
  Eff Map : Lookup_n-D  BreakpointsForDimension1=PlntEM1SpdEff*30/pi  BreakpointsForDimension2=PlntEM1TrqEff  Table=PlntEM1EffTbl  ExtrapMethod=Clip  UseLastTableValue=on  InternalRulePriority=Speed  OutDataTypeStr=Inherit: Inherit from 'Table data'  RndMeth=Simplest
      settings: InputPortMap=u0,u1
  Gain1 : Gain  Gain=1/100
  Math Function : Math  Operator=pow  SignedPower=on  OutputSignalType=real
  Product : Product
  Product3 : Product
  Product4 : Product
  Switch2 : Switch  SaturateOnIntegerOverflow=off  InputSameDT=off
  rads_to_rpm : Gain  Gain=30/pi
  MotPwrElecReq : Outport  VectorParamsAs1DForOutWhenUnconnected=off
  wires:
  Product3/1 -> Product4/1
  Switch2/1 -> Math Function/2
  Constant1/1 -> Switch2/1
  Constant2/1 -> Switch2/3
  Eff Map/1 -> Gain1/1
  Abs/1 -> Eff Map/1
  Gain1/1 -> Math Function/1
  Math Function/1 -> Product4/2
  Product4/1 -> MotPwrElecReq/1
  Abs1/1 -> Eff Map/2
  rads_to_rpm/1 -> Abs/1
  Product/1 -> Switch2/2
  MotSpd/1 -> Product3/1, Product/1, rads_to_rpm/1
  MotTrqCmd/1 -> Product3/2, Product/2, Abs1/1

== system HevMmPowertrainController/Multi-Mode_Hybrid_Control/ChargeSustain_Mode.Generator_Control.On.GenControl/State-Feedback Controller ==
  r : Inport
  y : Inport  Port=2
  Discrete-Time Integrator1 : DiscreteIntegrator  IntegratorMethod=Integration: Backward Euler  gainval=1  SampleTime=-1  ICPrevOutput=DiscIntNeverNeededParam  ICPrevScaledInput=DiscIntNeverNeededParam
  Gain1 : Gain  Gain=[3 -1]  Multiplication=Matrix(K*u)
  Mux1 : Mux  Inputs=2
  Saturation : Saturate  UpperLimit=max(PlntEM2Trq)  LowerLimit=-max(PlntEM2Trq)
  Sum : Sum  Inputs=|+-
  Out1 : Outport  VectorParamsAs1DForOutWhenUnconnected=off
  wires:
  Mux1/1 -> Gain1/1
  Discrete-Time Integrator1/1 -> Mux1/1
  Sum/1 -> Discrete-Time Integrator1/1  "err"
  r/1 -> Sum/1
  Gain1/1 -> Saturation/1
  y/1 -> Mux1/2, Sum/2
  Saturation/1 -> Out1/1

== system HevMmPowertrainController/Multi-Mode_Hybrid_Control/ChargeSustain_Mode.Generator_Control.On.GenControl/Torque Limit ==
  GenTrq : Inport
  GenSpd : Inport  Port=2
  Abs : Abs  SaturateOnIntegerOverflow=off
  Gain : Gain  Gain=-1
  GenMotTrqVsSpd : Lookup_n-D  NumberOfTableDimensions=1  BreakpointsForDimension1=PlntEM2Spd*30/pi  Table=PlntEM2Trq  ExtrapMethod=Clip  UseLastTableValue=on  InternalRulePriority=Speed  OutDataTypeStr=Inherit: Inherit from 'Table data'  RndMeth=Simplest
  Saturation Dynamic : simulink/Discontinuities/Saturation Dynamic  OutMin=[]  OutMax=[]  OutDataTypeStr=Inherit: Same as second input  OutDataType=fixdt(1, 16)  OutScaling=2^-10  DoSatur=off
  rads_to_rpm : Gain  Gain=30/pi
  GenTrqCmd : Outport  VectorParamsAs1DForOutWhenUnconnected=off
  wires:
  rads_to_rpm/1 -> GenMotTrqVsSpd/1
  Gain/1 -> Saturation Dynamic/3
  GenTrq/1 -> Saturation Dynamic/2
  Saturation Dynamic/1 -> GenTrqCmd/1
  GenSpd/1 -> Abs/1
  GenMotTrqVsSpd/1 -> Saturation Dynamic/1, Gain/1
  Abs/1 -> rads_to_rpm/1

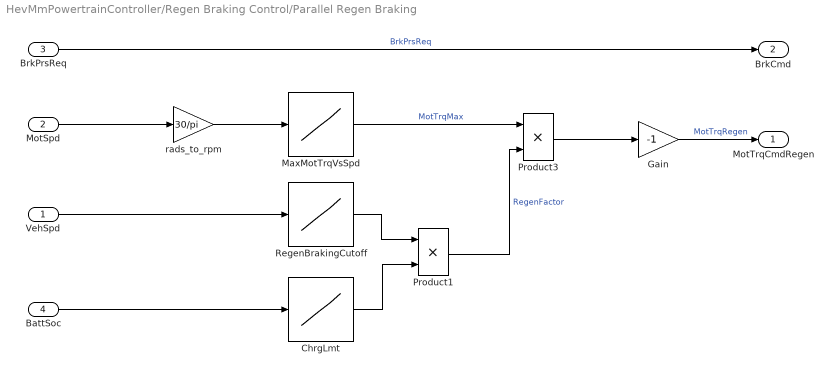
== system HevMmPowertrainController/Regen Braking Control/Parallel Regen Braking ==
  VehSpd : Inport
  "MotSpd " : Inport  Port=2
  "BrkPrsReq " : Inport  Port=3
  BattSoc : Inport  Port=4
  ChrgLmt : Lookup_n-D  NumberOfTableDimensions=1  BreakpointsForDimension1=CtrlVcuHevMmSocBpt  Table=CtrlVcuHevMmChrgLmtBpt  ExtrapMethod=Clip  UseLastTableValue=on  InternalRulePriority=Speed  RndMeth=Simplest
  Gain : Gain  Gain=-1
  MaxMotTrqVsSpd : Lookup_n-D  NumberOfTableDimensions=1  BreakpointsForDimension1=PlntEM1Spd*30/pi  Table=PlntEM1Trq  ExtrapMethod=Clip  UseLastTableValue=on  InternalRulePriority=Speed  OutDataTypeStr=Inherit: Inherit from 'Table data'  RndMeth=Simplest
  Product1 : Product
  Product3 : Product
  RegenBrakingCutoff : Lookup_n-D  NumberOfTableDimensions=1  BreakpointsForDimension1=CtrlVcuHevMmRegenBrkSpdBpt  Table=CtrlVcuHevMmRegenBrkCutOff  ExtrapMethod=Clip  UseLastTableValue=on  InternalRulePriority=Speed  RndMeth=Simplest
  rads_to_rpm : Gain  Gain=30/pi
  " MotTrqCmdRegen" : Outport  VectorParamsAs1DForOutWhenUnconnected=off
  " BrkCmd" : Outport  Port=2  VectorParamsAs1DForOutWhenUnconnected=off
  wires:
  Gain/1 -> " MotTrqCmdRegen"/1  "MotTrqRegen"
  BattSoc/1 -> ChrgLmt/1
  Product3/1 -> Gain/1
  Product1/1 -> Product3/2  "RegenFactor"
  RegenBrakingCutoff/1 -> Product1/1
  VehSpd/1 -> RegenBrakingCutoff/1
  ChrgLmt/1 -> Product1/2
  MaxMotTrqVsSpd/1 -> Product3/1  "MotTrqMax"
  rads_to_rpm/1 -> MaxMotTrqVsSpd/1
  "MotSpd "/1 -> rads_to_rpm/1
  "BrkPrsReq "/1 -> " BrkCmd"/1  "BrkPrsReq"

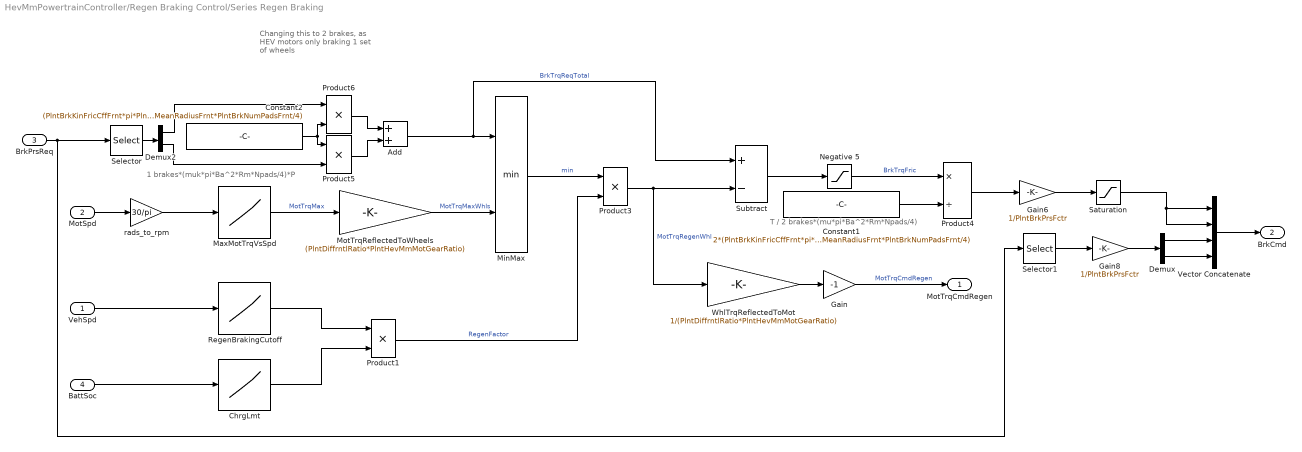
== system HevMmPowertrainController/Regen Braking Control/Series Regen Braking ==
  note: T / 2 brakes*(mu*pi*Ba^2*Rm*Npads/4)
  note: Changing this to 2 brakes,
      | as HEV motors only braking
      | 1 set of wheels
  note: 1 brakes*(muk*pi*Ba^2*Rm*Npads/4)*P
  VehSpd : Inport
  "MotSpd " : Inport  Port=2
  "BrkPrsReq " : Inport  Port=3
  BattSoc : Inport  Port=4
  Add : Sum
  ChrgLmt : Lookup_n-D  NumberOfTableDimensions=1  BreakpointsForDimension1=CtrlVcuHevMmSocBpt  Table=CtrlVcuHevMmChrgLmtBpt  ExtrapMethod=Clip  UseLastTableValue=on  InternalRulePriority=Speed  RndMeth=Simplest
  Constant1 : Constant  Value=2*(PlntBrkKinFricCffFrnt*pi*PlntBrkActrBoreFrnt^2*PlntBrkPadMeanRadiusFrnt*PlntBrkNumPadsFrnt/4)  SampleTime=-1
  Constant2 : Constant  Value=(PlntBrkKinFricCffFrnt*pi*PlntBrkActrBoreFrnt^2*PlntBrkPadMeanRadiusFrnt*PlntBrkNumPadsFrnt/4)  SampleTime=-1
  Demux : Demux  Outputs=2
  Demux2 : Demux  Outputs=2
  Gain : Gain  Gain=-1
  Gain6 : Gain  Gain=1/PlntBrkPrsFctr
  Gain8 : Gain  Gain=1/PlntBrkPrsFctr
  MaxMotTrqVsSpd : Lookup_n-D  NumberOfTableDimensions=1  BreakpointsForDimension1=PlntEM1Spd*30/pi  Table=PlntEM1Trq  ExtrapMethod=Clip  UseLastTableValue=on  InternalRulePriority=Speed  OutDataTypeStr=Inherit: Inherit from 'Table data'  RndMeth=Simplest
  MinMax : MinMax  Inputs=2
  MotTrqReflectedToWheels : Gain  Gain=(PlntDiffrntlRatio*PlntHevMmMotGearRatio)
  Negative 5 : Saturate  UpperLimit=inf  LowerLimit=0
  Product{1,3,5..6} (4 alike) : Product
  Product4 : Product  Inputs=*/
  RegenBrakingCutoff : Lookup_n-D  NumberOfTableDimensions=1  BreakpointsForDimension1=CtrlVcuHevMmRegenBrkSpdBpt  Table=CtrlVcuHevMmRegenBrkCutOff  ExtrapMethod=Clip  UseLastTableValue=on  InternalRulePriority=Speed  RndMeth=Simplest
  Saturation : Saturate  UpperLimit=1  LowerLimit=0
  Selector : Selector  InputPortWidth=4  IndexOptions=Index vector (dialog)  Indices=[1 2]  OutputSizes=1
  Selector1 : Selector  InputPortWidth=4  IndexOptions=Index vector (dialog)  Indices=[3 4]  OutputSizes=1
  Subtract : Sum  Inputs=+-
  Vector Concatenate : Concatenate  NumInputs=4
  WhlTrqReflectedToMot : Gain  Gain=1/(PlntDiffrntlRatio*PlntHevMmMotGearRatio)
  rads_to_rpm : Gain  Gain=30/pi
  " MotTrqCmdRegen" : Outport  VectorParamsAs1DForOutWhenUnconnected=off
  " BrkCmd" : Outport  Port=2  VectorParamsAs1DForOutWhenUnconnected=off
  wires:
  Product3/1 -> WhlTrqReflectedToMot/1, Subtract/2  "MotTrqRegenWhl"
  Constant1/1 -> Product4/2
  rads_to_rpm/1 -> MaxMotTrqVsSpd/1
  MaxMotTrqVsSpd/1 -> MotTrqReflectedToWheels/1  "MotTrqMax"
  MinMax/1 -> Product3/1  "min"
  ChrgLmt/1 -> Product1/2
  VehSpd/1 -> RegenBrakingCutoff/1
  RegenBrakingCutoff/1 -> Product1/1
  Product1/1 -> Product3/2  "RegenFactor"
  Subtract/1 -> Negative 5/1
  BattSoc/1 -> ChrgLmt/1
  Negative 5/1 -> Product4/1  "BrkTrqFric"
  "MotSpd "/1 -> rads_to_rpm/1
  MotTrqReflectedToWheels/1 -> MinMax/2  "MotTrqMaxWhls"
  WhlTrqReflectedToMot/1 -> Gain/1
  Gain/1 -> " MotTrqCmdRegen"/1  "MotTrqCmdRegen"
  Add/1 -> MinMax/1, Subtract/1  "BrkTrqReqTotal"
  Selector/1 -> Demux2/1
  Constant2/1 -> Product6/2, Product5/1
  Product6/1 -> Add/1
  Demux2/2 -> Product5/2
  Demux2/1 -> Product6/1
  Product5/1 -> Add/2
  Demux/2 -> Vector Concatenate/4
  Vector Concatenate/1 -> " BrkCmd"/1
  Demux/1 -> Vector Concatenate/3
  Saturation/1 -> Vector Concatenate/2, Vector Concatenate/1
  Gain6/1 -> Saturation/1
  "BrkPrsReq "/1 -> Selector1/1, Selector/1
  Selector1/1 -> Gain8/1
  Product4/1 -> Gain6/1
  Gain8/1 -> Demux/1

== system HevMmPowertrainController/Motor Torque Arbitration and Power Management/Power Management/Check Within Limits ==
  up : Inport
  u : Inport  Port=2
  lo : Inport  Port=3
  Compare To Zero : simulink/Logic and Bit Operations/Compare To Zero  relop=>=  OutDataTypeStr=boolean
  Compare To Zero1 : simulink/Logic and Bit Operations/Compare To Zero  relop=<=  OutDataTypeStr=boolean
  Logical Operator : Logic  AllPortsSameDT=off  OutDataTypeStr=boolean
  Saturation Dynamic1 : simulink/Discontinuities/Saturation Dynamic  OutMin=[]  OutMax=[]  OutDataTypeStr=Inherit: Same as second input  OutDataType=fixdt(1, 16)  OutScaling=2^-10  DoSatur=off
  Subtract : Sum  Inputs=+-
  Subtract1 : Sum  Inputs=-+
  InLimit : Outport  VectorParamsAs1DForOutWhenUnconnected=off
  y : Outport  Port=2  VectorParamsAs1DForOutWhenUnconnected=off
  wires:
  Saturation Dynamic1/1 -> y/1
  lo/1 -> Subtract1/2, Saturation Dynamic1/3
  up/1 -> Subtract/1, Saturation Dynamic1/1
  u/1 -> Subtract1/1, Subtract/2, Saturation Dynamic1/2
  Subtract/1 -> Compare To Zero/1
  Subtract1/1 -> Compare To Zero1/1
  Compare To Zero/1 -> Logical Operator/1
  Compare To Zero1/1 -> Logical Operator/2
  Logical Operator/1 -> InLimit/1

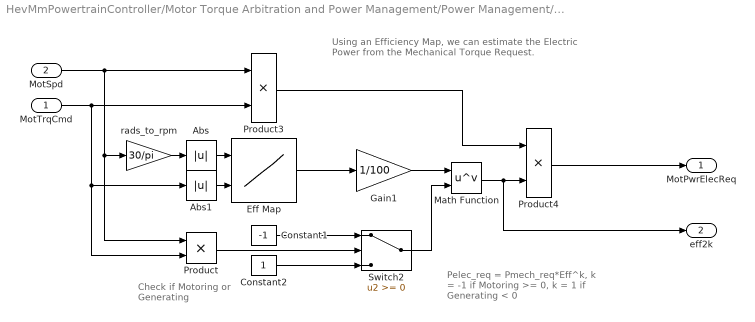
== system HevMmPowertrainController/Motor Torque Arbitration and Power Management/Power Management/Mech to Elec Power Estimate ==
  note: Check if Motoring
      | or Generating
  note: Using an Efficiency Map, we can estimate the
      | Electric Power from the Mechanical  Torque Request.
  note: Pelec_req = Pmech_req*Eff^k,
      | k = -1 if Motoring >= 0,
      | k = 1 if Generating < 0
  MotTrqCmd : Inport
  MotSpd : Inport  Port=2
  Abs : Abs  SaturateOnIntegerOverflow=off
  Abs1 : Abs  SaturateOnIntegerOverflow=off
  Constant1 : Constant  Value=-1  SampleTime=-1
  Constant2 : Constant  SampleTime=-1
  Eff Map : Lookup_n-D  BreakpointsForDimension1=PlntEM1SpdEff*30/pi  BreakpointsForDimension2=PlntEM1TrqEff  Table=PlntEM1EffTbl  ExtrapMethod=Clip  UseLastTableValue=on  InternalRulePriority=Speed  OutDataTypeStr=Inherit: Inherit from 'Table data'  RndMeth=Simplest
      settings: InputPortMap=u0,u1
  Gain1 : Gain  Gain=1/100
  Math Function : Math  Operator=pow  SignedPower=on  OutputSignalType=real
  Product : Product
  Product3 : Product
  Product4 : Product
  Switch2 : Switch  SaturateOnIntegerOverflow=off  InputSameDT=off
  rads_to_rpm : Gain  Gain=30/pi
  MotPwrElecReq : Outport  VectorParamsAs1DForOutWhenUnconnected=off
  eff2k : Outport  Port=2  VectorParamsAs1DForOutWhenUnconnected=off
  wires:
  Product3/1 -> Product4/1
  Switch2/1 -> Math Function/2
  Constant1/1 -> Switch2/1
  Constant2/1 -> Switch2/3
  Eff Map/1 -> Gain1/1
  Abs/1 -> Eff Map/1
  Gain1/1 -> Math Function/1
  Math Function/1 -> eff2k/1, Product4/2
  Product4/1 -> MotPwrElecReq/1
  Abs1/1 -> Eff Map/2
  rads_to_rpm/1 -> Abs/1
  Product/1 -> Switch2/2
  MotSpd/1 -> Product3/1, Product/1, rads_to_rpm/1
  MotTrqCmd/1 -> Product3/2, Product/2, Abs1/1

== system HevMmPowertrainController/Motor Torque Arbitration and Power Management/Power Management/Torque Limit ==
  MotTrq : Inport
  MotSpd : Inport  Port=2
  Gain : Gain  Gain=-1
  MaxMotTrqVsSpd : Lookup_n-D  NumberOfTableDimensions=1  BreakpointsForDimension1=PlntEM1Spd*30/pi  Table=PlntEM1Trq  ExtrapMethod=Clip  UseLastTableValue=on  InternalRulePriority=Speed  OutDataTypeStr=Inherit: Inherit from 'Table data'  RndMeth=Simplest
  Saturation Dynamic : simulink/Discontinuities/Saturation Dynamic  OutMin=[]  OutMax=[]  OutDataTypeStr=Inherit: Same as second input  OutDataType=fixdt(1, 16)  OutScaling=2^-10  DoSatur=off
  rads_to_rpm : Gain  Gain=30/pi
  MotTrqCmd : Outport  VectorParamsAs1DForOutWhenUnconnected=off
  wires:
  MotTrq/1 -> Saturation Dynamic/2
  Saturation Dynamic/1 -> MotTrqCmd/1
  MotSpd/1 -> rads_to_rpm/1
  MaxMotTrqVsSpd/1 -> Gain/1, Saturation Dynamic/1
  rads_to_rpm/1 -> MaxMotTrqVsSpd/1
  Gain/1 -> Saturation Dynamic/3
